simulink model "ccmotor"  (R2017a)
settings: Solver=VariableStepAuto  StartTime=0.0  StopTime=10.0  RelTol=1e-3
undefined symbols (not defined in the file): DiscIntNeverNeededParam
libraries: ccmotor_lib x1
settings Model: Creator=jdam  LastModifiedBy=jdam

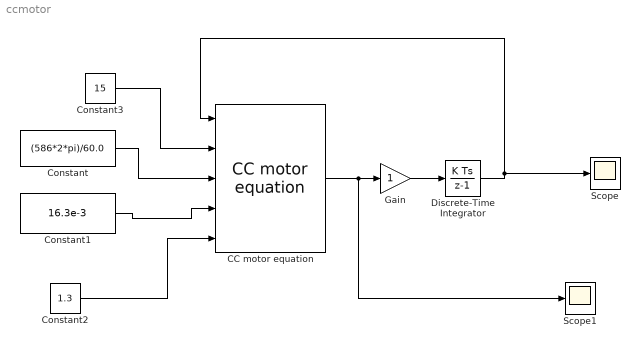
== system ccmotor ==
  CC motor equation : ccmotor_lib/CC motor equation
  Constant : Constant  Value=(586*2*pi)/60.0
  Constant1 : Constant  Value=16.3e-3
  Constant2 : Constant  Value=1.3
  Constant3 : Constant  Value=15
  Discrete-Time Integrator : DiscreteIntegrator  InitialConditionSetting=State (most efficient)  SampleTime=-1  ICPrevOutput=DiscIntNeverNeededParam  ICPrevScaledInput=DiscIntNeverNeededParam
  Gain : Gain
  Scope : Scope
  Scope1 : Scope
  wires:
  CC motor equation/1 -> Scope1/1, Gain/1
  Gain/1 -> Discrete-Time Integrator/1
  Discrete-Time Integrator/1 -> Scope/1, CC motor equation/1
  Constant/1 -> CC motor equation/3
  Constant1/1 -> CC motor equation/4
  Constant2/1 -> CC motor equation/5
  Constant3/1 -> CC motor equation/2
